simulink model "PhysicalHyperCook"  (R2026a)
settings: Solver=VariableStepAuto  StopTime=14400
undefined symbols (not defined in the file): Fault_T_Cook1, Fault_T_Cook2, Fault_T_Cook3, Fault_T_Cook4, Fault_T_Pack, Fault_T_Prep1, Fault_T_Prep2, Fault_T_QC, HC_PackRate_bph, HC_PrepRate_bph, HC_QCRate_bph, HC_Resupply_bph, Recipe_Block_s, Recipe_Count, Recipe_Flush_s, Resupply_Cutoff_T, Transport_Latency_s, Transport_Rate_bph
(part 2 of 2)

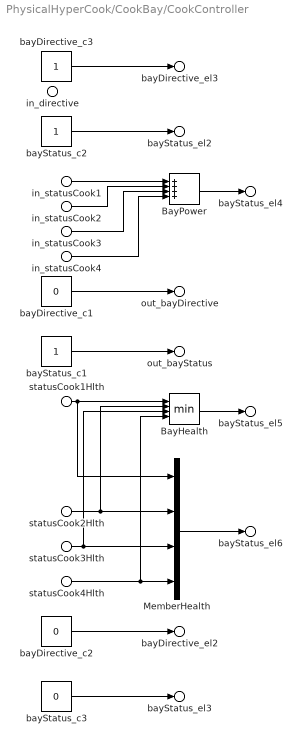
== system PhysicalHyperCook/CookBay/CookController ==
  in_directive : Inport  PortName=directive
  in_statusCook1 : Inport  Port=2  PortName=statusCook1  Element=power_kW
  statusCook1Hlth : Inport  Port=2  PortName=statusCook1  Element=health
  in_statusCook2 : Inport  Port=3  PortName=statusCook2  Element=power_kW
  statusCook2Hlth : Inport  Port=3  PortName=statusCook2  Element=health
  in_statusCook3 : Inport  Port=4  PortName=statusCook3  Element=power_kW
  statusCook3Hlth : Inport  Port=4  PortName=statusCook3  Element=health
  in_statusCook4 : Inport  Port=5  PortName=statusCook4  Element=power_kW
  statusCook4Hlth : Inport  Port=5  PortName=statusCook4  Element=health
  BayHealth : MinMax  Inputs=4
  BayPower : Sum  Inputs=++++
  MemberHealth : Mux
  bayDirective_c1 : Constant  Value=0
  bayDirective_c2 : Constant  Value=0
  bayDirective_c3 : Constant
  bayStatus_c1 : Constant
  bayStatus_c2 : Constant
  bayStatus_c3 : Constant  Value=0
  out_bayDirective : Outport  PortName=bayDirective  Element=cmdType
  bayDirective_el2 : Outport  PortName=bayDirective  Element=targetId
  bayDirective_el3 : Outport  PortName=bayDirective  Element=setpoint
  out_bayStatus : Outport  Port=2  PortName=bayStatus  Element=unitId
  bayStatus_el2 : Outport  Port=2  PortName=bayStatus  Element=opState
  bayStatus_el3 : Outport  Port=2  PortName=bayStatus  Element=faultCode
  bayStatus_el4 : Outport  Port=2  PortName=bayStatus  Element=power_kW
  bayStatus_el5 : Outport  Port=2  PortName=bayStatus  Element=health
  bayStatus_el6 : Outport  Port=2  PortName=bayStatus  Element=lineHealth
  wires:
  bayDirective_c3/1 -> bayDirective_el3/1
  bayStatus_c1/1 -> out_bayStatus/1
  bayStatus_c2/1 -> bayStatus_el2/1
  in_statusCook4/1 -> BayPower/4
  in_statusCook3/1 -> BayPower/3
  in_statusCook2/1 -> BayPower/2
  in_statusCook1/1 -> BayPower/1
  bayDirective_c1/1 -> out_bayDirective/1
  statusCook1Hlth/1 -> MemberHealth/1, BayHealth/1
  bayDirective_c2/1 -> bayDirective_el2/1
  statusCook2Hlth/1 -> BayHealth/2, MemberHealth/2
  statusCook3Hlth/1 -> BayHealth/3, MemberHealth/3
  statusCook4Hlth/1 -> BayHealth/4, MemberHealth/4
  BayPower/1 -> bayStatus_el4/1
  bayStatus_c3/1 -> bayStatus_el3/1
  BayHealth/1 -> bayStatus_el5/1
  MemberHealth/1 -> bayStatus_el6/1

== system PhysicalHyperCook/FinishingLine/FinishingController ==
  in_directive : Inport  PortName=directive
  in_statusPack : Inport  Port=2  PortName=statusPack  Element=power_kW
  statusPackHlth : Inport  Port=2  PortName=statusPack  Element=health
  in_statusQA : Inport  Port=3  PortName=statusQA  Element=power_kW
  statusQAHlth : Inport  Port=3  PortName=statusQA  Element=health
  BayHealth : MinMax  Inputs=2
  BayPower : Sum
  HealthPad : Constant
  MemberHealth : Mux
  bayDirective_c1 : Constant  Value=0
  bayDirective_c2 : Constant  Value=0
  bayDirective_c3 : Constant
  bayStatus_c1 : Constant
  bayStatus_c2 : Constant
  bayStatus_c3 : Constant  Value=0
  out_bayDirective : Outport  PortName=bayDirective  Element=cmdType
  bayDirective_el2 : Outport  PortName=bayDirective  Element=targetId
  bayDirective_el3 : Outport  PortName=bayDirective  Element=setpoint
  out_bayStatus : Outport  Port=2  PortName=bayStatus  Element=unitId
  bayStatus_el2 : Outport  Port=2  PortName=bayStatus  Element=opState
  bayStatus_el3 : Outport  Port=2  PortName=bayStatus  Element=faultCode
  bayStatus_el4 : Outport  Port=2  PortName=bayStatus  Element=power_kW
  bayStatus_el5 : Outport  Port=2  PortName=bayStatus  Element=health
  bayStatus_el6 : Outport  Port=2  PortName=bayStatus  Element=lineHealth
  wires:
  statusQAHlth/1 -> BayHealth/1, MemberHealth/1
  bayDirective_c3/1 -> bayDirective_el3/1
  bayStatus_c2/1 -> bayStatus_el2/1
  in_statusQA/1 -> BayPower/1
  bayStatus_c1/1 -> out_bayStatus/1
  bayDirective_c1/1 -> out_bayDirective/1
  in_statusPack/1 -> BayPower/2
  bayStatus_c3/1 -> bayStatus_el3/1
  BayPower/1 -> bayStatus_el4/1
  HealthPad/1 -> MemberHealth/3, MemberHealth/4
  statusPackHlth/1 -> BayHealth/2, MemberHealth/2
  bayDirective_c2/1 -> bayDirective_el2/1
  MemberHealth/1 -> bayStatus_el6/1
  BayHealth/1 -> bayStatus_el5/1

== system PhysicalHyperCook/FinishingLine/HighSpeedPackagingLine ==
  in_approvedSoup : Inport  PortName=approvedSoup  Element=flow_bps
  in_directive : Inport  Port=2  PortName=directive  Element=setpoint
  En_Gate_Fault_T_Pack : Product
  Gate_Fault_T_Pack : Step  Time=Fault_T_Pack  InitialValue=1  FinalValue=0  SampleTime=0
  NoBehaviorsModeled : Subsystem
  Pack : ModelReference  ModelNameDialog=BehPackager  UsingDefaultArgumentValue=0,0  SimulationMode=Normal  ModelReferenceVersion=1.5
  PackDraw : Constant  Value=HC_PackRate_bph/3600
  Surge : ModelReference  ModelNameDialog=BehStorage  UsingDefaultArgumentValue=0,0  SimulationMode=Normal  ModelReferenceVersion=1.4
  Trm13 : Terminator
  Trm14 : Terminator
  out_sealedContainers : Outport  PortName=sealedContainers  Element=batchId
  sealedContainers_el2 : Outport  PortName=sealedContainers  Element=count
  sealedContainers_el3 : Outport  PortName=sealedContainers  Element=sealRating_days
  sealedContainers_el4 : Outport  PortName=sealedContainers  Element=flow_bps
  out_statusPack : Outport  Port=2  PortName=statusPack  Element=unitId
  statusPack_el2 : Outport  Port=2  PortName=statusPack  Element=opState
  statusPack_el3 : Outport  Port=2  PortName=statusPack  Element=faultCode
  statusPack_el4 : Outport  Port=2  PortName=statusPack  Element=power_kW
  statusPack_el5 : Outport  Port=2  PortName=statusPack  Element=health
  wires:
  Surge/3 -> Trm14/1
  Surge/1 -> Pack/1
  PackDraw/1 -> Surge/2
  Pack/1 -> sealedContainers_el4/1
  in_directive/1 -> En_Gate_Fault_T_Pack/1
  Gate_Fault_T_Pack/1 -> statusPack_el5/1, En_Gate_Fault_T_Pack/2
  in_approvedSoup/1 -> Surge/1
  En_Gate_Fault_T_Pack/1 -> Pack/2
  Surge/2 -> Trm13/1
  NoBehaviorsModeled/1(Out1) -> out_sealedContainers/1
  NoBehaviorsModeled/2(Out2) -> sealedContainers_el2/1
  NoBehaviorsModeled/3(Out3) -> sealedContainers_el3/1
  NoBehaviorsModeled/4(Out4) -> statusPack_el2/1
  NoBehaviorsModeled/5(Out5) -> statusPack_el3/1
  NoBehaviorsModeled/6(Out6) -> statusPack_el4/1
  NoBehaviorsModeled/7(Out7) -> out_statusPack/1

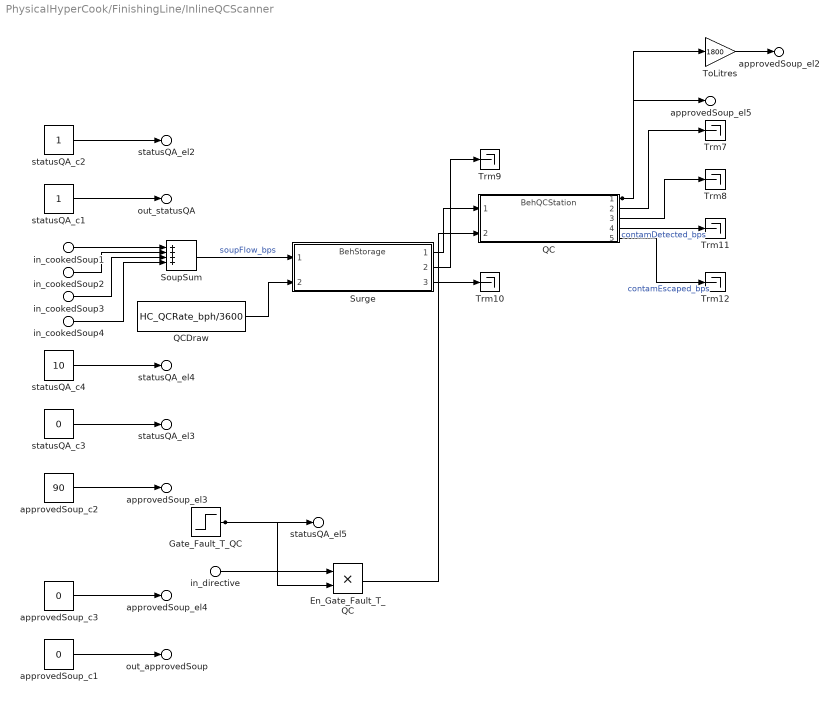
== system PhysicalHyperCook/FinishingLine/InlineQCScanner ==
  in_cookedSoup1 : Inport  PortName=cookedSoup1  Element=flow_bps
  in_cookedSoup2 : Inport  Port=2  PortName=cookedSoup2  Element=flow_bps
  in_cookedSoup3 : Inport  Port=3  PortName=cookedSoup3  Element=flow_bps
  in_cookedSoup4 : Inport  Port=4  PortName=cookedSoup4  Element=flow_bps
  in_directive : Inport  Port=5  PortName=directive  Element=setpoint
  En_Gate_Fault_T_QC : Product
  Gate_Fault_T_QC : Step  Time=Fault_T_QC  InitialValue=1  FinalValue=0  SampleTime=0
  QC : ModelReference  ModelNameDialog=BehQCStation  UsingDefaultArgumentValue=0,0,0,0,0,0  SimulationMode=Normal  ModelReferenceVersion=1.6
  QCDraw : Constant  Value=HC_QCRate_bph/3600
  SoupSum : Sum  Inputs=++++
  Surge : ModelReference  ModelNameDialog=BehStorage  UsingDefaultArgumentValue=0,0  SimulationMode=Normal  ModelReferenceVersion=1.4
  ToLitres : Gain  Gain=1800
  Trm{7..12} (6 alike) : Terminator
  approvedSoup_c1 : Constant  Value=0
  approvedSoup_c2 : Constant  Value=90
  approvedSoup_c3 : Constant  Value=0
  statusQA_c1 : Constant
  statusQA_c2 : Constant
  statusQA_c3 : Constant  Value=0
  statusQA_c4 : Constant  Value=10
  out_approvedSoup : Outport  PortName=approvedSoup  Element=batchId
  approvedSoup_el2 : Outport  PortName=approvedSoup  Element=volume_L
  approvedSoup_el3 : Outport  PortName=approvedSoup  Element=temp_C
  approvedSoup_el4 : Outport  PortName=approvedSoup  Element=contamination_ppm
  approvedSoup_el5 : Outport  PortName=approvedSoup  Element=flow_bps
  out_statusQA : Outport  Port=2  PortName=statusQA  Element=unitId
  statusQA_el2 : Outport  Port=2  PortName=statusQA  Element=opState
  statusQA_el3 : Outport  Port=2  PortName=statusQA  Element=faultCode
  statusQA_el4 : Outport  Port=2  PortName=statusQA  Element=power_kW
  statusQA_el5 : Outport  Port=2  PortName=statusQA  Element=health
  wires:
  statusQA_c4/1 -> statusQA_el4/1
  approvedSoup_c3/1 -> approvedSoup_el4/1
  statusQA_c2/1 -> statusQA_el2/1
  Gate_Fault_T_QC/1 -> En_Gate_Fault_T_QC/2, statusQA_el5/1
  statusQA_c3/1 -> statusQA_el3/1
  in_cookedSoup4/1 -> SoupSum/4
  statusQA_c1/1 -> out_statusQA/1
  in_cookedSoup1/1 -> SoupSum/1
  in_cookedSoup2/1 -> SoupSum/2
  in_cookedSoup3/1 -> SoupSum/3
  approvedSoup_c2/1 -> approvedSoup_el3/1
  ToLitres/1 -> approvedSoup_el2/1
  approvedSoup_c1/1 -> out_approvedSoup/1
  En_Gate_Fault_T_QC/1 -> QC/2
  SoupSum/1 -> Surge/1  "soupFlow_bps"
  QCDraw/1 -> Surge/2
  in_directive/1 -> En_Gate_Fault_T_QC/1
  Surge/1 -> QC/1
  Surge/2 -> Trm9/1
  QC/2 -> Trm7/1
  Surge/3 -> Trm10/1
  QC/1 -> ToLitres/1, approvedSoup_el5/1
  QC/3 -> Trm8/1
  QC/4 -> Trm11/1  "contamDetected_bps"
  QC/5 -> Trm12/1  "contamEscaped_bps"

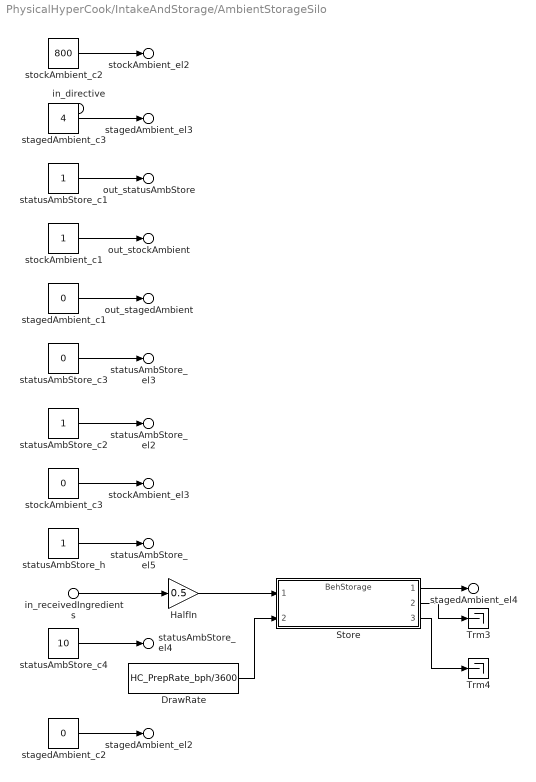
== system PhysicalHyperCook/IntakeAndStorage/AmbientStorageSilo ==
  in_receivedIngredients : Inport  PortName=receivedIngredients  Element=flow_bps
  in_directive : Inport  Port=2  PortName=directive  Element=setpoint
  DrawRate : Constant  Value=HC_PrepRate_bph/3600
  HalfIn : Gain  Gain=0.5
  Store : ModelReference  ModelNameDialog=BehStorage  UsingDefaultArgumentValue=0,0  SimulationMode=Normal  ModelReferenceVersion=1.4
  Trm3 : Terminator
  Trm4 : Terminator
  stagedAmbient_c1 : Constant  Value=0
  stagedAmbient_c2 : Constant  Value=0
  stagedAmbient_c3 : Constant  Value=4
  statusAmbStore_c1 : Constant
  statusAmbStore_c2 : Constant
  statusAmbStore_c3 : Constant  Value=0
  statusAmbStore_c4 : Constant  Value=10
  statusAmbStore_h : Constant
  stockAmbient_c1 : Constant
  stockAmbient_c2 : Constant  Value=800
  stockAmbient_c3 : Constant  Value=0
  out_stagedAmbient : Outport  PortName=stagedAmbient  Element=palletId
  stagedAmbient_el2 : Outport  PortName=stagedAmbient  Element=mass_kg
  stagedAmbient_el3 : Outport  PortName=stagedAmbient  Element=temp_C
  stagedAmbient_el4 : Outport  PortName=stagedAmbient  Element=flow_bps
  out_stockAmbient : Outport  Port=2  PortName=stockAmbient  Element=itemId
  stockAmbient_el2 : Outport  Port=2  PortName=stockAmbient  Element=qty_units
  stockAmbient_el3 : Outport  Port=2  PortName=stockAmbient  Element=error_pct
  out_statusAmbStore : Outport  Port=3  PortName=statusAmbStore  Element=unitId
  statusAmbStore_el2 : Outport  Port=3  PortName=statusAmbStore  Element=opState
  statusAmbStore_el3 : Outport  Port=3  PortName=statusAmbStore  Element=faultCode
  statusAmbStore_el4 : Outport  Port=3  PortName=statusAmbStore  Element=power_kW
  statusAmbStore_el5 : Outport  Port=3  PortName=statusAmbStore  Element=health
  wires:
  statusAmbStore_c1/1 -> out_statusAmbStore/1
  stockAmbient_c2/1 -> stockAmbient_el2/1
  Store/3 -> Trm4/1
  stockAmbient_c3/1 -> stockAmbient_el3/1
  Store/1 -> stagedAmbient_el4/1
  statusAmbStore_c2/1 -> statusAmbStore_el2/1
  stagedAmbient_c1/1 -> out_stagedAmbient/1
  stockAmbient_c1/1 -> out_stockAmbient/1
  stagedAmbient_c3/1 -> stagedAmbient_el3/1
  statusAmbStore_c3/1 -> statusAmbStore_el3/1
  statusAmbStore_h/1 -> statusAmbStore_el5/1
  in_receivedIngredients/1 -> HalfIn/1
  statusAmbStore_c4/1 -> statusAmbStore_el4/1
  stagedAmbient_c2/1 -> stagedAmbient_el2/1
  HalfIn/1 -> Store/1
  DrawRate/1 -> Store/2
  Store/2 -> Trm3/1

== system PhysicalHyperCook/IntakeAndStorage/CargoGantryDock ==
  in_inboundCargo : Inport  PortName=inboundCargo  Element=flow_bps
  in_directive : Inport  Port=2  PortName=directive
  in_inboundCargoCap : Saturate  UpperLimit=0.111111111111  LowerLimit=0
  receivedIngredients_c1 : Constant  Value=0
  receivedIngredients_c2 : Constant  Value=0
  receivedIngredients_c3 : Constant  Value=4
  statusReceive_c1 : Constant
  statusReceive_c2 : Constant
  statusReceive_c3 : Constant  Value=0
  statusReceive_c4 : Constant  Value=15
  statusReceive_h : Constant
  out_receivedIngredients : Outport  PortName=receivedIngredients  Element=palletId
  receivedIngredients_el2 : Outport  PortName=receivedIngredients  Element=mass_kg
  receivedIngredients_el3 : Outport  PortName=receivedIngredients  Element=temp_C
  receivedIngredients_el4 : Outport  PortName=receivedIngredients  Element=flow_bps
  out_statusReceive : Outport  Port=2  PortName=statusReceive  Element=unitId
  statusReceive_el2 : Outport  Port=2  PortName=statusReceive  Element=opState
  statusReceive_el3 : Outport  Port=2  PortName=statusReceive  Element=faultCode
  statusReceive_el4 : Outport  Port=2  PortName=statusReceive  Element=power_kW
  statusReceive_el5 : Outport  Port=2  PortName=statusReceive  Element=health
  wires:
  receivedIngredients_c1/1 -> out_receivedIngredients/1
  receivedIngredients_c3/1 -> receivedIngredients_el3/1
  statusReceive_c1/1 -> out_statusReceive/1
  statusReceive_c4/1 -> statusReceive_el4/1
  statusReceive_h/1 -> statusReceive_el5/1
  receivedIngredients_c2/1 -> receivedIngredients_el2/1
  statusReceive_c2/1 -> statusReceive_el2/1
  in_inboundCargo/1 -> in_inboundCargoCap/1
  statusReceive_c3/1 -> statusReceive_el3/1
  in_inboundCargoCap/1 -> receivedIngredients_el4/1

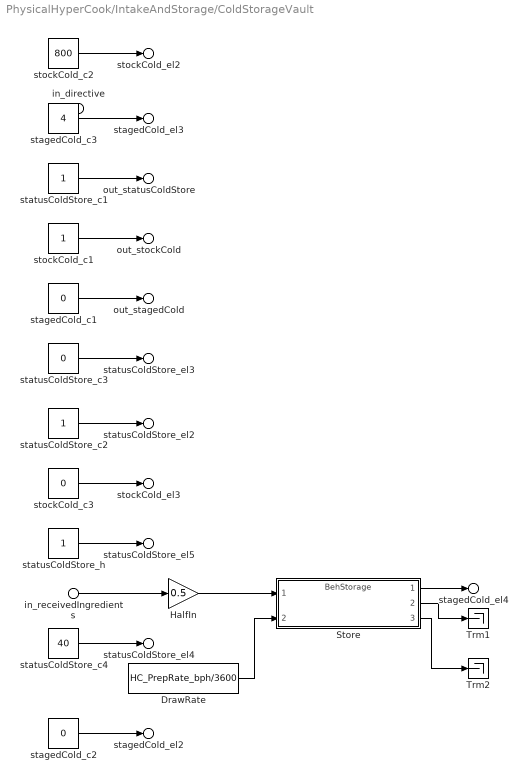
== system PhysicalHyperCook/IntakeAndStorage/ColdStorageVault ==
  in_receivedIngredients : Inport  PortName=receivedIngredients  Element=flow_bps
  in_directive : Inport  Port=2  PortName=directive  Element=setpoint
  DrawRate : Constant  Value=HC_PrepRate_bph/3600
  HalfIn : Gain  Gain=0.5
  Store : ModelReference  ModelNameDialog=BehStorage  UsingDefaultArgumentValue=0,0  SimulationMode=Normal  ModelReferenceVersion=1.4
  Trm1 : Terminator
  Trm2 : Terminator
  stagedCold_c1 : Constant  Value=0
  stagedCold_c2 : Constant  Value=0
  stagedCold_c3 : Constant  Value=4
  statusColdStore_c1 : Constant
  statusColdStore_c2 : Constant
  statusColdStore_c3 : Constant  Value=0
  statusColdStore_c4 : Constant  Value=40
  statusColdStore_h : Constant
  stockCold_c1 : Constant
  stockCold_c2 : Constant  Value=800
  stockCold_c3 : Constant  Value=0
  out_stagedCold : Outport  PortName=stagedCold  Element=palletId
  stagedCold_el2 : Outport  PortName=stagedCold  Element=mass_kg
  stagedCold_el3 : Outport  PortName=stagedCold  Element=temp_C
  stagedCold_el4 : Outport  PortName=stagedCold  Element=flow_bps
  out_stockCold : Outport  Port=2  PortName=stockCold  Element=itemId
  stockCold_el2 : Outport  Port=2  PortName=stockCold  Element=qty_units
  stockCold_el3 : Outport  Port=2  PortName=stockCold  Element=error_pct
  out_statusColdStore : Outport  Port=3  PortName=statusColdStore  Element=unitId
  statusColdStore_el2 : Outport  Port=3  PortName=statusColdStore  Element=opState
  statusColdStore_el3 : Outport  Port=3  PortName=statusColdStore  Element=faultCode
  statusColdStore_el4 : Outport  Port=3  PortName=statusColdStore  Element=power_kW
  statusColdStore_el5 : Outport  Port=3  PortName=statusColdStore  Element=health
  wires:
  statusColdStore_c3/1 -> statusColdStore_el3/1
  statusColdStore_c1/1 -> out_statusColdStore/1
  stockCold_c2/1 -> stockCold_el2/1
  stockCold_c3/1 -> stockCold_el3/1
  statusColdStore_c2/1 -> statusColdStore_el2/1
  stagedCold_c1/1 -> out_stagedCold/1
  stockCold_c1/1 -> out_stockCold/1
  stagedCold_c3/1 -> stagedCold_el3/1
  stagedCold_c2/1 -> stagedCold_el2/1
  statusColdStore_h/1 -> statusColdStore_el5/1
  in_receivedIngredients/1 -> HalfIn/1
  statusColdStore_c4/1 -> statusColdStore_el4/1
  HalfIn/1 -> Store/1
  DrawRate/1 -> Store/2
  Store/1 -> stagedCold_el4/1
  Store/2 -> Trm1/1
  Store/3 -> Trm2/1

== system PhysicalHyperCook/IntakeAndStorage/IntakeController ==
  in_directive : Inport  PortName=directive
  in_statusAmbStore : Inport  Port=2  PortName=statusAmbStore  Element=power_kW
  statusAmbStoreHlth : Inport  Port=2  PortName=statusAmbStore  Element=health
  in_statusReceive : Inport  Port=3  PortName=statusReceive  Element=power_kW
  statusReceiveHlth : Inport  Port=3  PortName=statusReceive  Element=health
  in_statusColdStore : Inport  Port=4  PortName=statusColdStore  Element=power_kW
  statusColdStoreHlth : Inport  Port=4  PortName=statusColdStore  Element=health
  BayHealth : MinMax  Inputs=3
  BayPower : Sum  Inputs=+++
  HealthPad : Constant
  MemberHealth : Mux
  bayDirective_c1 : Constant  Value=0
  bayDirective_c2 : Constant  Value=0
  bayDirective_c3 : Constant
  bayStatus_c1 : Constant
  bayStatus_c2 : Constant
  bayStatus_c3 : Constant  Value=0
  out_bayDirective : Outport  PortName=bayDirective  Element=cmdType
  bayDirective_el2 : Outport  PortName=bayDirective  Element=targetId
  bayDirective_el3 : Outport  PortName=bayDirective  Element=setpoint
  out_bayStatus : Outport  Port=2  PortName=bayStatus  Element=unitId
  bayStatus_el2 : Outport  Port=2  PortName=bayStatus  Element=opState
  bayStatus_el3 : Outport  Port=2  PortName=bayStatus  Element=faultCode
  bayStatus_el4 : Outport  Port=2  PortName=bayStatus  Element=power_kW
  bayStatus_el5 : Outport  Port=2  PortName=bayStatus  Element=health
  bayStatus_el6 : Outport  Port=2  PortName=bayStatus  Element=lineHealth
  wires:
  bayStatus_c3/1 -> bayStatus_el3/1
  in_statusColdStore/1 -> BayPower/2
  in_statusAmbStore/1 -> BayPower/3
  in_statusReceive/1 -> BayPower/1
  bayStatus_c1/1 -> out_bayStatus/1
  BayPower/1 -> bayStatus_el4/1
  bayStatus_c2/1 -> bayStatus_el2/1
  bayDirective_c3/1 -> bayDirective_el3/1
  bayDirective_c1/1 -> out_bayDirective/1
  statusAmbStoreHlth/1 -> BayHealth/3, MemberHealth/3
  statusReceiveHlth/1 -> BayHealth/1, MemberHealth/1
  HealthPad/1 -> MemberHealth/4
  statusColdStoreHlth/1 -> BayHealth/2, MemberHealth/2
  bayDirective_c2/1 -> bayDirective_el2/1
  MemberHealth/1 -> bayStatus_el6/1
  BayHealth/1 -> bayStatus_el5/1

== system PhysicalHyperCook/IntakeAndStorage/InventorySensorGrid ==
  in_stockCold : Inport  PortName=stockCold
  in_stockAmbient : Inport  Port=2  PortName=stockAmbient
  inventoryStatus_c1 : Constant
  inventoryStatus_c2 : Constant  Value=800
  inventoryStatus_c3 : Constant  Value=0
  reorderRequest_c1 : Constant
  reorderRequest_c2 : Constant  Value=0
  reorderRequest_c3 : Constant  Value=0
  out_inventoryStatus : Outport  PortName=inventoryStatus  Element=itemId
  inventoryStatus_el2 : Outport  PortName=inventoryStatus  Element=qty_units
  inventoryStatus_el3 : Outport  PortName=inventoryStatus  Element=error_pct
  out_reorderRequest : Outport  Port=2  PortName=reorderRequest  Element=itemId
  reorderRequest_el2 : Outport  Port=2  PortName=reorderRequest  Element=qty_units
  reorderRequest_el3 : Outport  Port=2  PortName=reorderRequest  Element=error_pct
  wires:
  reorderRequest_c3/1 -> reorderRequest_el3/1
  reorderRequest_c2/1 -> reorderRequest_el2/1
  inventoryStatus_c2/1 -> inventoryStatus_el2/1
  inventoryStatus_c3/1 -> inventoryStatus_el3/1
  inventoryStatus_c1/1 -> out_inventoryStatus/1
  reorderRequest_c1/1 -> out_reorderRequest/1

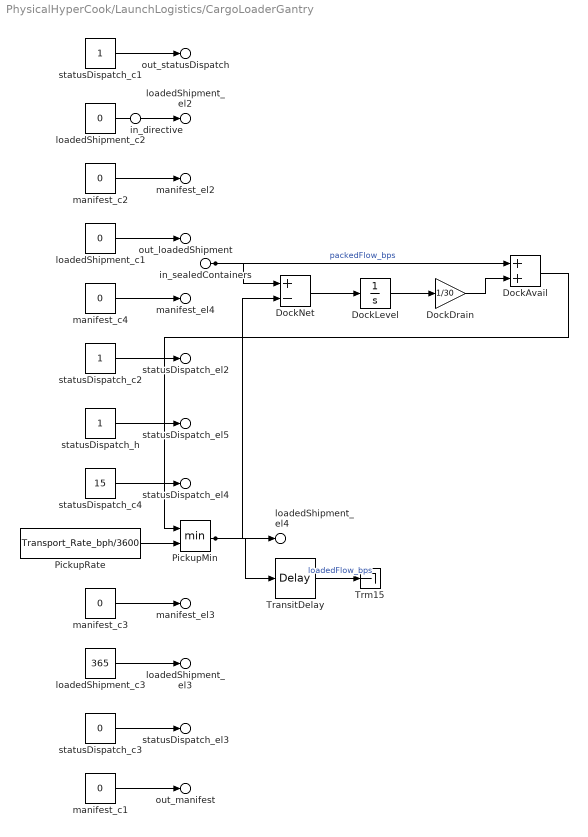
== system PhysicalHyperCook/LaunchLogistics/CargoLoaderGantry ==
  in_sealedContainers : Inport  PortName=sealedContainers  Element=flow_bps
  in_directive : Inport  Port=2  PortName=directive
  DockAvail : Sum
  DockDrain : Gain  Gain=1/30
  DockLevel : Integrator  LimitOutput=on  UpperSaturationLimit=600  LowerSaturationLimit=0
  DockNet : Sum  Inputs=+-
  PickupMin : MinMax  Inputs=2
  PickupRate : Constant  Value=Transport_Rate_bph/3600
  TransitDelay : TransportDelay  DelayTime=Transport_Latency_s
  Trm15 : Terminator
  loadedShipment_c1 : Constant  Value=0
  loadedShipment_c2 : Constant  Value=0
  loadedShipment_c3 : Constant  Value=365
  manifest_c{1..4} (4 alike) : Constant  Value=0
  statusDispatch_c1 : Constant
  statusDispatch_c2 : Constant
  statusDispatch_c3 : Constant  Value=0
  statusDispatch_c4 : Constant  Value=15
  statusDispatch_h : Constant
  out_loadedShipment : Outport  PortName=loadedShipment  Element=batchId
  loadedShipment_el2 : Outport  PortName=loadedShipment  Element=count
  loadedShipment_el3 : Outport  PortName=loadedShipment  Element=sealRating_days
  loadedShipment_el4 : Outport  PortName=loadedShipment  Element=flow_bps
  out_manifest : Outport  Port=2  PortName=manifest  Element=destinationId
  manifest_el2 : Outport  Port=2  PortName=manifest  Element=batchId
  manifest_el3 : Outport  Port=2  PortName=manifest  Element=count
  manifest_el4 : Outport  Port=2  PortName=manifest  Element=mass_kg
  out_statusDispatch : Outport  Port=3  PortName=statusDispatch  Element=unitId
  statusDispatch_el2 : Outport  Port=3  PortName=statusDispatch  Element=opState
  statusDispatch_el3 : Outport  Port=3  PortName=statusDispatch  Element=faultCode
  statusDispatch_el4 : Outport  Port=3  PortName=statusDispatch  Element=power_kW
  statusDispatch_el5 : Outport  Port=3  PortName=statusDispatch  Element=health
  wires:
  manifest_c4/1 -> manifest_el4/1
  manifest_c2/1 -> manifest_el2/1
  statusDispatch_c1/1 -> out_statusDispatch/1
  DockAvail/1 -> PickupMin/1
  loadedShipment_c1/1 -> out_loadedShipment/1
  DockNet/1 -> DockLevel/1
  loadedShipment_c2/1 -> loadedShipment_el2/1
  statusDispatch_c3/1 -> statusDispatch_el3/1
  statusDispatch_h/1 -> statusDispatch_el5/1
  manifest_c1/1 -> out_manifest/1
  statusDispatch_c2/1 -> statusDispatch_el2/1
  statusDispatch_c4/1 -> statusDispatch_el4/1
  PickupRate/1 -> PickupMin/2
  manifest_c3/1 -> manifest_el3/1
  loadedShipment_c3/1 -> loadedShipment_el3/1
  in_sealedContainers/1 -> DockAvail/1, DockNet/1  "packedFlow_bps"
  PickupMin/1 -> DockNet/2, loadedShipment_el4/1, TransitDelay/1
  TransitDelay/1 -> Trm15/1  "loadedFlow_bps"
  DockLevel/1 -> DockDrain/1
  DockDrain/1 -> DockAvail/2

== system PhysicalHyperCook/LaunchLogistics/LaunchController ==
  in_directive : Inport  PortName=directive
  in_statusDispatch : Inport  Port=2  PortName=statusDispatch  Element=power_kW
  statusDispatchHlth : Inport  Port=2  PortName=statusDispatch  Element=health
  in_statusFleet : Inport  Port=3  PortName=statusFleet  Element=power_kW
  statusFleetHlth : Inport  Port=3  PortName=statusFleet  Element=health
  in_statusRefuel : Inport  Port=4  PortName=statusRefuel  Element=power_kW
  statusRefuelHlth : Inport  Port=4  PortName=statusRefuel  Element=health
  BayHealth : MinMax  Inputs=3
  BayPower : Sum  Inputs=+++
  HealthPad : Constant
  MemberHealth : Mux
  bayDirective_c1 : Constant  Value=0
  bayDirective_c2 : Constant  Value=0
  bayDirective_c3 : Constant
  bayStatus_c1 : Constant
  bayStatus_c2 : Constant
  bayStatus_c3 : Constant  Value=0
  out_bayDirective : Outport  PortName=bayDirective  Element=cmdType
  bayDirective_el2 : Outport  PortName=bayDirective  Element=targetId
  bayDirective_el3 : Outport  PortName=bayDirective  Element=setpoint
  out_bayStatus : Outport  Port=2  PortName=bayStatus  Element=unitId
  bayStatus_el2 : Outport  Port=2  PortName=bayStatus  Element=opState
  bayStatus_el3 : Outport  Port=2  PortName=bayStatus  Element=faultCode
  bayStatus_el4 : Outport  Port=2  PortName=bayStatus  Element=power_kW
  bayStatus_el5 : Outport  Port=2  PortName=bayStatus  Element=health
  bayStatus_el6 : Outport  Port=2  PortName=bayStatus  Element=lineHealth
  wires:
  bayStatus_c3/1 -> bayStatus_el3/1
  bayStatus_c1/1 -> out_bayStatus/1
  BayPower/1 -> bayStatus_el4/1
  bayStatus_c2/1 -> bayStatus_el2/1
  bayDirective_c1/1 -> out_bayDirective/1
  bayDirective_c3/1 -> bayDirective_el3/1
  in_statusDispatch/1 -> BayPower/1
  in_statusRefuel/1 -> BayPower/3
  in_statusFleet/1 -> BayPower/2
  statusRefuelHlth/1 -> BayHealth/3, MemberHealth/3
  statusDispatchHlth/1 -> BayHealth/1, MemberHealth/1
  HealthPad/1 -> MemberHealth/4
  statusFleetHlth/1 -> MemberHealth/2, BayHealth/2
  bayDirective_c2/1 -> bayDirective_el2/1
  MemberHealth/1 -> bayStatus_el6/1
  BayHealth/1 -> bayStatus_el5/1

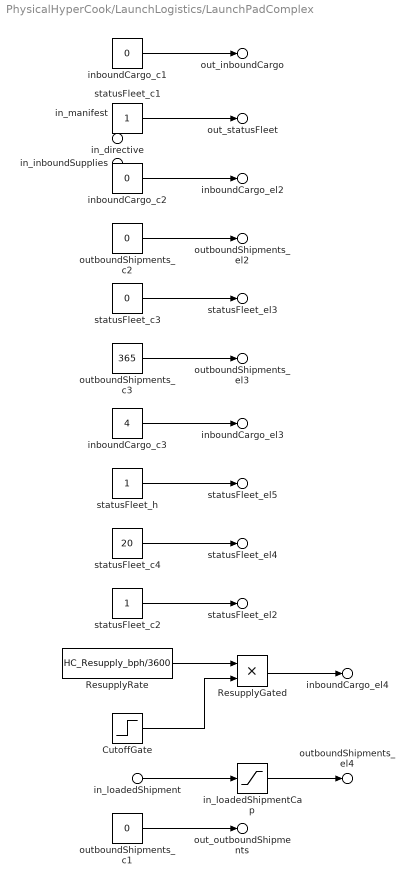
== system PhysicalHyperCook/LaunchLogistics/LaunchPadComplex ==
  in_loadedShipment : Inport  PortName=loadedShipment  Element=flow_bps
  in_manifest : Inport  Port=2  PortName=manifest
  in_directive : Inport  Port=3  PortName=directive
  in_inboundSupplies : Inport  Port=4  PortName=inboundSupplies
  CutoffGate : Step  Time=Resupply_Cutoff_T  InitialValue=1  FinalValue=0  SampleTime=0
  ResupplyGated : Product
  ResupplyRate : Constant  Value=HC_Resupply_bph/3600
  in_loadedShipmentCap : Saturate  UpperLimit=0.1  LowerLimit=0
  inboundCargo_c1 : Constant  Value=0
  inboundCargo_c2 : Constant  Value=0
  inboundCargo_c3 : Constant  Value=4
  outboundShipments_c1 : Constant  Value=0
  outboundShipments_c2 : Constant  Value=0
  outboundShipments_c3 : Constant  Value=365
  statusFleet_c1 : Constant
  statusFleet_c2 : Constant
  statusFleet_c3 : Constant  Value=0
  statusFleet_c4 : Constant  Value=20
  statusFleet_h : Constant
  out_inboundCargo : Outport  PortName=inboundCargo  Element=palletId
  inboundCargo_el2 : Outport  PortName=inboundCargo  Element=mass_kg
  inboundCargo_el3 : Outport  PortName=inboundCargo  Element=temp_C
  inboundCargo_el4 : Outport  PortName=inboundCargo  Element=flow_bps
  out_outboundShipments : Outport  Port=2  PortName=outboundShipments  Element=batchId
  outboundShipments_el2 : Outport  Port=2  PortName=outboundShipments  Element=count
  outboundShipments_el3 : Outport  Port=2  PortName=outboundShipments  Element=sealRating_days
  outboundShipments_el4 : Outport  Port=2  PortName=outboundShipments  Element=flow_bps
  out_statusFleet : Outport  Port=3  PortName=statusFleet  Element=unitId
  statusFleet_el2 : Outport  Port=3  PortName=statusFleet  Element=opState
  statusFleet_el3 : Outport  Port=3  PortName=statusFleet  Element=faultCode
  statusFleet_el4 : Outport  Port=3  PortName=statusFleet  Element=power_kW
  statusFleet_el5 : Outport  Port=3  PortName=statusFleet  Element=health
  wires:
  inboundCargo_c1/1 -> out_inboundCargo/1
  in_loadedShipmentCap/1 -> outboundShipments_el4/1
  CutoffGate/1 -> ResupplyGated/2
  statusFleet_h/1 -> statusFleet_el5/1
  statusFleet_c3/1 -> statusFleet_el3/1
  inboundCargo_c3/1 -> inboundCargo_el3/1
  inboundCargo_c2/1 -> inboundCargo_el2/1
  ResupplyGated/1 -> inboundCargo_el4/1
  statusFleet_c1/1 -> out_statusFleet/1
  in_loadedShipment/1 -> in_loadedShipmentCap/1
  outboundShipments_c2/1 -> outboundShipments_el2/1
  outboundShipments_c3/1 -> outboundShipments_el3/1
  statusFleet_c4/1 -> statusFleet_el4/1
  statusFleet_c2/1 -> statusFleet_el2/1
  ResupplyRate/1 -> ResupplyGated/1
  outboundShipments_c1/1 -> out_outboundShipments/1

== system PhysicalHyperCook/LaunchLogistics/RefuelingStation ==
  in_directive : Inport  PortName=directive
  statusRefuel_c1 : Constant
  statusRefuel_c2 : Constant
  statusRefuel_c3 : Constant  Value=0
  statusRefuel_c4 : Constant  Value=20
  statusRefuel_h : Constant
  out_statusRefuel : Outport  PortName=statusRefuel  Element=unitId
  statusRefuel_el2 : Outport  PortName=statusRefuel  Element=opState
  statusRefuel_el3 : Outport  PortName=statusRefuel  Element=faultCode
  statusRefuel_el4 : Outport  PortName=statusRefuel  Element=power_kW
  statusRefuel_el5 : Outport  PortName=statusRefuel  Element=health
  wires:
  statusRefuel_h/1 -> statusRefuel_el5/1
  statusRefuel_c3/1 -> statusRefuel_el3/1
  statusRefuel_c1/1 -> out_statusRefuel/1
  statusRefuel_c2/1 -> statusRefuel_el2/1
  statusRefuel_c4/1 -> statusRefuel_el4/1

== system PhysicalHyperCook/PlantServices/ConveyorNetwork ==
  in_transportDirective : Inport  PortName=transportDirective
  statusTransport_c1 : Constant
  statusTransport_c2 : Constant
  statusTransport_c3 : Constant  Value=0
  statusTransport_c4 : Constant  Value=25
  statusTransport_h : Constant
  out_statusTransport : Outport  PortName=statusTransport  Element=unitId
  statusTransport_el2 : Outport  PortName=statusTransport  Element=opState
  statusTransport_el3 : Outport  PortName=statusTransport  Element=faultCode
  statusTransport_el4 : Outport  PortName=statusTransport  Element=power_kW
  statusTransport_el5 : Outport  PortName=statusTransport  Element=health
  wires:
  statusTransport_h/1 -> statusTransport_el5/1
  statusTransport_c3/1 -> statusTransport_el3/1
  statusTransport_c1/1 -> out_statusTransport/1
  statusTransport_c2/1 -> statusTransport_el2/1
  statusTransport_c4/1 -> statusTransport_el4/1

== system PhysicalHyperCook/PlantServices/FusionPowerPlant ==
  in_directive : Inport  PortName=directive
  statusPower_c1 : Constant
  statusPower_c2 : Constant
  statusPower_c3 : Constant  Value=0
  statusPower_c4 : Constant  Value=0
  statusPower_h : Constant
  out_statusPower : Outport  PortName=statusPower  Element=unitId
  statusPower_el2 : Outport  PortName=statusPower  Element=opState
  statusPower_el3 : Outport  PortName=statusPower  Element=faultCode
  statusPower_el4 : Outport  PortName=statusPower  Element=power_kW
  statusPower_el5 : Outport  PortName=statusPower  Element=health
  wires:
  statusPower_h/1 -> statusPower_el5/1
  statusPower_c3/1 -> statusPower_el3/1
  statusPower_c1/1 -> out_statusPower/1
  statusPower_c2/1 -> statusPower_el2/1
  statusPower_c4/1 -> statusPower_el4/1

== system PhysicalHyperCook/PlantServices/GravityCompensatorArray ==
  in_ambientGravity : Inport  PortName=ambientGravity  Element=gravity_g
  envStatus_c1 : Constant  Value=100
  out_envStatus : Outport  PortName=envStatus  Element=gravity_g
  envStatus_el2 : Outport  PortName=envStatus  Element=compensation_pct
  wires:
  envStatus_c1/1 -> envStatus_el2/1
  in_ambientGravity/1 -> out_envStatus/1  "ambientGravity"

== system PhysicalHyperCook/PlantServices/ServicesController ==
  in_directive : Inport  PortName=directive
  in_statusTransport : Inport  Port=2  PortName=statusTransport  Element=power_kW
  statusTransportHlth : Inport  Port=2  PortName=statusTransport  Element=health
  in_statusPower : Inport  Port=3  PortName=statusPower  Element=power_kW
  statusPowerHlth : Inport  Port=3  PortName=statusPower  Element=health
  BayHealth : MinMax  Inputs=2
  BayPower : Sum
  HealthPad : Constant
  MemberHealth : Mux
  bayDirective_c1 : Constant  Value=0
  bayDirective_c2 : Constant  Value=0
  bayDirective_c3 : Constant
  bayStatus_c1 : Constant
  bayStatus_c2 : Constant
  bayStatus_c3 : Constant  Value=0
  out_bayDirective : Outport  PortName=bayDirective  Element=cmdType
  bayDirective_el2 : Outport  PortName=bayDirective  Element=targetId
  bayDirective_el3 : Outport  PortName=bayDirective  Element=setpoint
  out_bayStatus : Outport  Port=2  PortName=bayStatus  Element=unitId
  bayStatus_el2 : Outport  Port=2  PortName=bayStatus  Element=opState
  bayStatus_el3 : Outport  Port=2  PortName=bayStatus  Element=faultCode
  bayStatus_el4 : Outport  Port=2  PortName=bayStatus  Element=power_kW
  bayStatus_el5 : Outport  Port=2  PortName=bayStatus  Element=health
  bayStatus_el6 : Outport  Port=2  PortName=bayStatus  Element=lineHealth
  wires:
  BayHealth/1 -> bayStatus_el5/1
  bayStatus_c2/1 -> bayStatus_el2/1
  bayDirective_c3/1 -> bayDirective_el3/1
  bayStatus_c1/1 -> out_bayStatus/1
  statusPowerHlth/1 -> BayHealth/1, MemberHealth/1
  in_statusTransport/1 -> BayPower/2
  bayStatus_c3/1 -> bayStatus_el3/1
  in_statusPower/1 -> BayPower/1
  bayDirective_c1/1 -> out_bayDirective/1
  HealthPad/1 -> MemberHealth/3, MemberHealth/4
  statusTransportHlth/1 -> BayHealth/2, MemberHealth/2
  bayDirective_c2/1 -> bayDirective_el2/1
  BayPower/1 -> bayStatus_el4/1
  MemberHealth/1 -> bayStatus_el6/1

== system PhysicalHyperCook/PrepBay/PrepController ==
  in_directive : Inport  PortName=directive
  in_statusPrep1 : Inport  Port=2  PortName=statusPrep1  Element=power_kW
  statusPrep1Hlth : Inport  Port=2  PortName=statusPrep1  Element=health
  in_statusPrep2 : Inport  Port=3  PortName=statusPrep2  Element=power_kW
  statusPrep2Hlth : Inport  Port=3  PortName=statusPrep2  Element=health
  BayHealth : MinMax  Inputs=2
  BayPower : Sum
  HealthPad : Constant
  MemberHealth : Mux
  bayDirective_c1 : Constant  Value=0
  bayDirective_c2 : Constant  Value=0
  bayDirective_c3 : Constant
  bayStatus_c1 : Constant
  bayStatus_c2 : Constant
  bayStatus_c3 : Constant  Value=0
  out_bayDirective : Outport  PortName=bayDirective  Element=cmdType
  bayDirective_el2 : Outport  PortName=bayDirective  Element=targetId
  bayDirective_el3 : Outport  PortName=bayDirective  Element=setpoint
  out_bayStatus : Outport  Port=2  PortName=bayStatus  Element=unitId
  bayStatus_el2 : Outport  Port=2  PortName=bayStatus  Element=opState
  bayStatus_el3 : Outport  Port=2  PortName=bayStatus  Element=faultCode
  bayStatus_el4 : Outport  Port=2  PortName=bayStatus  Element=power_kW
  bayStatus_el5 : Outport  Port=2  PortName=bayStatus  Element=health
  bayStatus_el6 : Outport  Port=2  PortName=bayStatus  Element=lineHealth
  wires:
  bayDirective_c1/1 -> out_bayDirective/1
  BayHealth/1 -> bayStatus_el5/1
  bayStatus_c2/1 -> bayStatus_el2/1
  statusPrep1Hlth/1 -> BayHealth/1, MemberHealth/1
  in_statusPrep2/1 -> BayPower/2
  in_statusPrep1/1 -> BayPower/1
  bayDirective_c3/1 -> bayDirective_el3/1
  bayStatus_c3/1 -> bayStatus_el3/1
  bayStatus_c1/1 -> out_bayStatus/1
  HealthPad/1 -> MemberHealth/3, MemberHealth/4
  statusPrep2Hlth/1 -> BayHealth/2, MemberHealth/2
  bayDirective_c2/1 -> bayDirective_el2/1
  BayPower/1 -> bayStatus_el4/1
  MemberHealth/1 -> bayStatus_el6/1

== system PhysicalHyperCook/PrepBay/RoboticPrepLine1 ==
  in_stagedCold : Inport  PortName=stagedCold  Element=flow_bps
  in_directive : Inport  Port=2  PortName=directive  Element=setpoint
  BlockFloor : Rounding
  BlockIndex : Gain  Gain=1/Recipe_Block_s
  En_Gate_Fault_T_Prep1 : Product
  Gate_Fault_T_Prep1 : Step  Time=Fault_T_Prep1  InitialValue=1  FinalValue=0  SampleTime=0
  Prep : ModelReference  ModelNameDialog=BehPrepUnit  UsingDefaultArgumentValue=0,0  SimulationMode=Normal  ModelReferenceVersion=1.5
  RecipeBias : Bias  Bias=1  SaturateOnIntegerOverflow=off
  RecipeClock : Clock
  RecipeCount : Constant  Value=Recipe_Count
  RecipeMod : Math  Operator=mod
  ToKgPerHr : Gain  Gain=0.55*3600
  Trm5 : Terminator
  preppedBatch1_c1 : Constant  Value=0
  statusPrep1_c1 : Constant
  statusPrep1_c2 : Constant
  statusPrep1_c3 : Constant  Value=0
  statusPrep1_c4 : Constant  Value=25
  out_preppedBatch1 : Outport  PortName=preppedBatch1  Element=batchId
  preppedBatch1_el2 : Outport  PortName=preppedBatch1  Element=recipeId
  preppedBatch1_el3 : Outport  PortName=preppedBatch1  Element=mass_kg
  preppedBatch1_el4 : Outport  PortName=preppedBatch1  Element=flow_bps
  out_statusPrep1 : Outport  Port=2  PortName=statusPrep1  Element=unitId
  statusPrep1_el2 : Outport  Port=2  PortName=statusPrep1  Element=opState
  statusPrep1_el3 : Outport  Port=2  PortName=statusPrep1  Element=faultCode
  statusPrep1_el4 : Outport  Port=2  PortName=statusPrep1  Element=power_kW
  statusPrep1_el5 : Outport  Port=2  PortName=statusPrep1  Element=health
  wires:
  statusPrep1_c1/1 -> out_statusPrep1/1
  statusPrep1_c4/1 -> statusPrep1_el4/1
  preppedBatch1_c1/1 -> out_preppedBatch1/1
  Gate_Fault_T_Prep1/1 -> En_Gate_Fault_T_Prep1/2, statusPrep1_el5/1
  statusPrep1_c3/1 -> statusPrep1_el3/1
  Prep/1 -> preppedBatch1_el4/1, ToKgPerHr/1
  statusPrep1_c2/1 -> statusPrep1_el2/1
  RecipeClock/1 -> BlockIndex/1
  RecipeBias/1 -> preppedBatch1_el2/1  "activeRecipe"
  in_directive/1 -> En_Gate_Fault_T_Prep1/1
  in_stagedCold/1 -> Prep/1
  En_Gate_Fault_T_Prep1/1 -> Prep/2
  BlockIndex/1 -> BlockFloor/1
  BlockFloor/1 -> RecipeMod/1
  Prep/2 -> Trm5/1
  RecipeCount/1 -> RecipeMod/2
  ToKgPerHr/1 -> preppedBatch1_el3/1
  RecipeMod/1 -> RecipeBias/1

== system PhysicalHyperCook/PrepBay/RoboticPrepLine2 ==
  in_stagedAmbient : Inport  PortName=stagedAmbient  Element=flow_bps
  in_directive : Inport  Port=2  PortName=directive  Element=setpoint
  BlockFloor : Rounding
  BlockIndex : Gain  Gain=1/Recipe_Block_s
  En_Gate_Fault_T_Prep2 : Product
  Gate_Fault_T_Prep2 : Step  Time=Fault_T_Prep2  InitialValue=1  FinalValue=0  SampleTime=0
  Prep : ModelReference  ModelNameDialog=BehPrepUnit  UsingDefaultArgumentValue=0,0  SimulationMode=Normal  ModelReferenceVersion=1.5
  RecipeBias : Bias  Bias=1  SaturateOnIntegerOverflow=off
  RecipeClock : Clock
  RecipeCount : Constant  Value=Recipe_Count
  RecipeMod : Math  Operator=mod
  ToKgPerHr : Gain  Gain=0.55*3600
  Trm6 : Terminator
  preppedBatch2_c1 : Constant  Value=0
  statusPrep2_c1 : Constant
  statusPrep2_c2 : Constant
  statusPrep2_c3 : Constant  Value=0
  statusPrep2_c4 : Constant  Value=25
  out_preppedBatch2 : Outport  PortName=preppedBatch2  Element=batchId
  preppedBatch2_el2 : Outport  PortName=preppedBatch2  Element=recipeId
  preppedBatch2_el3 : Outport  PortName=preppedBatch2  Element=mass_kg
  preppedBatch2_el4 : Outport  PortName=preppedBatch2  Element=flow_bps
  out_statusPrep2 : Outport  Port=2  PortName=statusPrep2  Element=unitId
  statusPrep2_el2 : Outport  Port=2  PortName=statusPrep2  Element=opState
  statusPrep2_el3 : Outport  Port=2  PortName=statusPrep2  Element=faultCode
  statusPrep2_el4 : Outport  Port=2  PortName=statusPrep2  Element=power_kW
  statusPrep2_el5 : Outport  Port=2  PortName=statusPrep2  Element=health
  wires:
  statusPrep2_c1/1 -> out_statusPrep2/1
  preppedBatch2_c1/1 -> out_preppedBatch2/1
  statusPrep2_c3/1 -> statusPrep2_el3/1
  RecipeClock/1 -> BlockIndex/1
  in_directive/1 -> En_Gate_Fault_T_Prep2/1
  Gate_Fault_T_Prep2/1 -> En_Gate_Fault_T_Prep2/2, statusPrep2_el5/1
  statusPrep2_c4/1 -> statusPrep2_el4/1
  statusPrep2_c2/1 -> statusPrep2_el2/1
  in_stagedAmbient/1 -> Prep/1
  En_Gate_Fault_T_Prep2/1 -> Prep/2
  Prep/2 -> Trm6/1
  BlockIndex/1 -> BlockFloor/1
  Prep/1 -> preppedBatch2_el4/1, ToKgPerHr/1
  BlockFloor/1 -> RecipeMod/1
  RecipeCount/1 -> RecipeMod/2
  ToKgPerHr/1 -> preppedBatch2_el3/1
  RecipeMod/1 -> RecipeBias/1
  RecipeBias/1 -> preppedBatch2_el2/1

== system PhysicalHyperCook/FinishingLine/HighSpeedPackagingLine/NoBehaviorsModeled ==
  note: No behaviors modeled
  sealedContainers_c1 : Constant  Value=0
  sealedContainers_c2 : Constant  Value=0
  sealedContainers_c3 : Constant  Value=365
  statusPack_c1 : Constant
  statusPack_c2 : Constant
  statusPack_c3 : Constant  Value=0
  statusPack_c4 : Constant  Value=35
  Out1 : Outport
  Out2 : Outport  Port=2
  Out3 : Outport  Port=3
  Out4 : Outport  Port=4
  Out5 : Outport  Port=5
  Out6 : Outport  Port=6
  Out7 : Outport  Port=7
  wires:
  sealedContainers_c2/1 -> Out2/1
  sealedContainers_c1/1 -> Out1/1
  statusPack_c4/1 -> Out6/1
  sealedContainers_c3/1 -> Out3/1
  statusPack_c1/1 -> Out7/1
  statusPack_c3/1 -> Out5/1
  statusPack_c2/1 -> Out4/1
